simulink model "Model_6DOF_B3"  (R2020b)
settings: Solver=FixedStepAuto  StartTime=0.0  StopTime=120  FixedStep=0.05  RelTol=1e-3
values from neighbouring files (symbols this model uses):
  Ba_0 = [0 0 0 0 0 0]    [ctrl_mode_param.m]
  Bb = 4418825.3321    [load_data.m]
  Bv_0 = [tgt_speed 0 0 0 0 0]    [ctrl_mode_param.m]
  Bx_0 = [0 0 tgt_depth 0 0 0]    [ctrl_mode_param.m]
  Ixx = 5.23e7    (= 52300000)    [load_data.m]
  Ixy = 0    [load_data.m]
  Ixz = 0    [load_data.m]
  Iyy = 1.375e9    (= 1375000000)    [load_data.m]
  Iyz = 0    [load_data.m]
  Izz = 1.367e9    (= 1367000000)    [load_data.m]
  Mb = 4418825.3321    [load_data.m]
  Xb = 0    [load_data.m]
  Xg = 0    [load_data.m]
  Yb = 0    [load_data.m]
  Yg = 0    [load_data.m]
  Zb = 0.4406    [load_data.m]
  Zg = 0    [load_data.m]
undefined symbols (not defined in the file or in its folder): dA_BP1, dA_BP2, dA_Hull, dA_PH, dA_Sail, dA_SProot, dA_X1a, dA_X1b, dA_X2a, dA_X2b, dA_X3a, dA_X3b, dA_X4a, dA_X4b, its, n_BP1, n_BP2, n_Hull, n_PH, n_Sail, n_SProot, n_X1a, n_X1b, n_X2a, n_X2b, n_X3a, n_X3b, n_X4a, n_X4b, nt_BP1, nt_BP2, nt_Hull, nt_PH, nt_Sail, nt_SProot, nt_X1a, nt_X1b, nt_X2a, nt_X2b, nt_X3a, nt_X3b, nt_X4a, nt_X4b, Usp, vt1_BP1, vt1_BP2, vt1_Hull, vt1_PH, vt1_Sail, vt1_SProot, vt1_X1a, vt1_X1b, vt1_X2a, vt1_X2b, vt1_X3a, vt1_X3b, vt1_X4a, vt1_X4b, vt2_BP1, vt2_BP2 ... (+27)
libraries: simulink x5
(part 11 of 15)

== matlab function Model_6DOF_B3/HDM B3/Wave, Virtual Mass and Hydrostatic/Wave Particle Motions/Subsystem/Subsystem/MATLAB Function4 ==
  data: time input; Xearth input; Fx_total output; vert1 input; vert2 input; vert3 input; dA input; ntri input; normal input; A_wave input; k_wave input; w_wave input; rho input; g input; Fy_total output; Fz_total output; Mx_total output; My_total output; Mz_total output; Zb input; its input; fwrite input
function [Fx_total,Fy_total,Fz_total,Mx_total,My_total,Mz_total]= fcn(time,Xearth,vert1,vert2,vert3,dA,ntri,normal,A_wave,k_wave,w_wave,rho,g,Zb,its,fwrite)
x_e=Xearth(1); y_e=Xearth(2); z_e=Xearth(3);
phi=Xearth(4); theta=Xearth(5); psi=Xearth(6);

RMat=[cos(theta)*cos(psi) -cos(phi)*sin(psi)+sin(phi)*sin(theta)*cos(psi)  sin(phi)*sin(psi)+cos(phi)*sin(theta)*cos(psi); ...
      cos(theta)*sin(psi)  cos(phi)*cos(psi)+sin(phi)*sin(theta)*sin(psi) -sin(phi)*cos(psi)+cos(phi)*sin(theta)*sin(psi); ...
     -sin(theta)                             sin(phi)*cos(theta)                             cos(phi)*cos(theta)];  

%position of mid points in earth coordinate;
mp1=zeros(ntri,3);
mp2=zeros(ntri,3);
mp3=zeros(ntri,3);
nA =zeros(ntri,3);

P1=zeros(ntri,1);
P2=zeros(ntri,1);
P3=zeros(ntri,1);

%position vector of mid points from the CG
r1=zeros(ntri,3);
r2=zeros(ntri,3);
r3=zeros(ntri,3);
v1_w=zeros(ntri,3);
v2_w=zeros(ntri,3);
v3_w=zeros(ntri,3);
n_w=zeros(ntri,3);

%Area of triangle, product of area and unit normal, position vector to each mid-point
for i=1:ntri
    %Area of each triangle
    A=[vert2(i,1)-vert1(i,1); vert2(i,2)-vert1(i,2); vert2(i,3)-vert1(i,3);];
    B=[vert3(i,1)-vert1(i,1); vert3(i,2)-vert1(i,2); vert3(i,3)-vert1(i,3);];
    C=[normal(i,1); normal(i,2); normal(i,3);];
        
    %A*n vector calculation
    for j=1:3
        nA(i,j)=dA(i).*C(j);    
    end
    
    %position vector to each mid point of each edge
    for j=1:3
        r1(i,j)=0.5*(vert1(i,j)+vert2(i,j));
        r2(i,j)=0.5*(vert1(i,j)+vert3(i,j));
        r3(i,j)=0.5*(vert2(i,j)+vert3(i,j));
    end
end

%computing mid point location between vertices in earth coordinate
for i=1:ntri
    MP1=RMat*[r1(i,1); r1(i,2); r1(i,3);]+[x_e; y_e; z_e;];
    MP2=RMat*[r2(i,1); r2(i,2); r2(i,3);]+[x_e; y_e; z_e;];
    MP3=RMat*[r3(i,1); r3(i,2); r3(i,3);]+[x_e; y_e; z_e;];
    
    v1i=RMat*[vert1(i,1); vert1(i,2); vert1(i,3);]+[x_e; y_e; z_e;];
    v2i=RMat*[vert2(i,1); vert2(i,2); vert2(i,3);]+[x_e; y_e; z_e;];
    v3i=RMat*[vert3(i,1); vert3(i,2); vert3(i,3);]+[x_e; y_e; z_e;];
   
    for j=1:3
        v1_w(i,j)=v1i(j); v2_w(i,j)=v2i(j); v3_w(i,j)=v3i(j); 
        mp1(i,j)=MP1(j);  mp2(i,j)=MP2(j);  mp3(i,j)=MP3(j);
    end
end

for i=1:ntri
    A=[v2_w(i,1)-v1_w(i,1); v2_w(i,2)-v1_w(i,2); v2_w(i,3)-v1_w(i,3);];
    B=[v3_w(i,1)-v1_w(i,1); v3_w(i,2)-v1_w(i,2); v3_w(i,3)-v1_w(i,3);];
    n=cross(A,B)/norm(cross(A,B));
    dA(i,1)=0.5*norm(cross(A,B));
    n_w(i,1)=n(1); n_w(i,2)=n(2); n_w(i,3)=n(3);
end

if fwrite==1
if rem(time,its)==0
%writing the transformed surface grid
filename=['./SurfOut/Hull_' sprintf('%08.2f',time) '.stl'];
fileID = fopen(filename,'w');
formatSpec='solid\n'; fprintf(fileID,formatSpec);
for i=1:ntri
fprintf(fileID,'facet normal ');
formatSpec='%1.8e %1.8e %1.8e\n';
fprintf(fileID,formatSpec,normal(i,1),normal(i,2),normal(i,3));
    fprintf(fileID,'  outer loop\n')
    fprintf(fileID,'    vertex   ')
    fprintf(fileID,formatSpec,v1_w(i,1)/70.2,v1_w(i,2)/70.2,v1_w(i,3)/70.2)
    fprintf(fileID,'    vertex   ')
    fprintf(fileID,formatSpec,v2_w(i,1)/70.2,v2_w(i,2)/70.2,v2_w(i,3)/70.2)
    fprintf(fileID,'    vertex   ')
    fprintf(fileID,formatSpec,v3_w(i,1)/70.2,v3_w(i,2)/70.2,v3_w(i,3)/70.2)
    fprintf(fileID,'  endloop\n')
    fprintf(fileID,'endfacet\n')
end
formatSpec='endsolid'; fprintf(fileID,formatSpec);
fclose(fileID);
end
end

%computing forces and moments for each triangle
Fx_total=0; Fy_total=0; Fz_total=0;
Mx_total=0; My_total=0; Mz_total=0;

for i=1:ntri
    p1=-rho*g*(mp1(i,3)-A_wave*exp(k_wave.*mp1(i,3)).*sin(k_wave*mp1(i,1)-w_wave.*time));
    p2=-rho*g*(mp2(i,3)-A_wave*exp(k_wave.*mp2(i,3)).*sin(k_wave*mp2(i,1)-w_wave.*time));
    p3=-rho*g*(mp3(i,3)-A_wave*exp(k_wave.*mp3(i,3)).*sin(k_wave*mp3(i,1)-w_wave.*time));
    
    dFx=-nA(i,1)*(p1+p2+p3)./3;
    dFy=-nA(i,2)*(p1+p2+p3)./3;
    dFz=-nA(i,3)*(p1+p2+p3)./3;
    
    dP =-p1.*[r1(i,1); r1(i,2); r1(i,3)-Zb;]...
        -p2.*[r2(i,1); r2(i,2); r2(i,3)-Zb;]...
        -p3.*[r3(i,1); r3(i,2); r3(i,3)-Zb;];
    N =[nA(i,1); nA(i,2); nA(i,3);];
    dM=cross(dP,N);
    Fx_total=Fx_total+dFx;
    Fy_total=Fy_total+dFy;
    Fz_total=Fz_total+dFz;
    Mx_total=Mx_total+dM(1)/3;
    My_total=My_total+dM(2)/3;
    Mz_total=Mz_total+dM(3)/3;
end
end

== matlab function Model_6DOF_B3/HDM B3/Wave, Virtual Mass and Hydrostatic/Wave Particle Motions/Subsystem/X1/MATLAB Function1 ==
  data: time input; Xearth input; Fx_total output; vert1 input; vert2 input; vert3 input; dA input; ntri input; normal input; A_wave input; k_wave input; w_wave input; rho input; g input; Fy_total output; Fz_total output; Mx_total output; My_total output; Mz_total output; Zb input; EAX input; dX input; its input; origin input; xcg input; fwrite input
function [Fx_total,Fy_total,Fz_total,Mx_total,My_total,Mz_total]= fcn(time,Xearth,vert1,vert2,vert3,dA,ntri,normal,A_wave,k_wave,w_wave,rho,g,Zb,EAX,dX,its,origin,xcg,fwrite)
%EAX=Appendage eulater angle in local coordinate
%its=number of time steps to skip writing grid

x_e=Xearth(1); y_e=Xearth(2); z_e=Xearth(3);
phi=Xearth(4); theta=Xearth(5); psi=Xearth(6);
phiX=EAX(1); thetaX=EAX(2); psiX=EAX(3);


RMat=[cos(theta)*cos(psi) -cos(phi)*sin(psi)+sin(phi)*sin(theta)*cos(psi)  sin(phi)*sin(psi)+cos(phi)*sin(theta)*cos(psi); ...
      cos(theta)*sin(psi)  cos(phi)*cos(psi)+sin(phi)*sin(theta)*sin(psi) -sin(phi)*cos(psi)+cos(phi)*sin(theta)*sin(psi); ...
     -sin(theta)                             sin(phi)*cos(theta)                             cos(phi)*cos(theta)];  
RMATX=[cos(thetaX)*cos(psiX) -cos(phiX)*sin(psiX)+sin(phiX)*sin(thetaX)*cos(psiX)  sin(phiX)*sin(psiX)+cos(phiX)*sin(thetaX)*cos(psiX); ...
      cos(thetaX)*sin(psiX)  cos(phiX)*cos(psiX)+sin(phiX)*sin(thetaX)*sin(psiX) -sin(phiX)*cos(psiX)+cos(phiX)*sin(thetaX)*sin(psiX); ...
     -sin(thetaX)                             sin(phiX)*cos(thetaX)                             cos(phiX)*cos(thetaX)];  
RMATD=[cos(0)*cos(dX) -cos(0)*sin(dX)+sin(0)*sin(0)*cos(dX)  sin(0)*sin(dX)+cos(0)*sin(0)*cos(dX); ...
      cos(0)*sin(dX)  cos(0)*cos(dX)+sin(0)*sin(0)*sin(dX) -sin(0)*cos(dX)+cos(0)*sin(0)*sin(dX); ...
     -sin(0)                             sin(0)*cos(0)                             cos(0)*cos(0)];  


%Rotating the vertices to put in ship coordinate
for i=1:ntri 
    V1=[vert1(i,1); vert1(i,2); vert1(i,3);];
    V2=[vert2(i,1); vert2(i,2); vert2(i,3);];
    V3=[vert3(i,1); vert3(i,2); vert3(i,3);];
        
    %rotating to local z coordinate
    V1_o=inv(RMATX)*(V1-origin*70.2+xcg);
    V2_o=inv(RMATX)*(V2-origin*70.2+xcg);
    V3_o=inv(RMATX)*(V3-origin*70.2+xcg);
    
    %rotating for corresponding appendage deflection
    V1_x=RMATD*V1_o;
    V2_x=RMATD*V2_o;
    V3_x=RMATD*V3_o;
    
        %re-positioning the appendage to local vectors
    V1_r=RMATX*V1_x;
    V2_r=RMATX*V2_x;
    V3_r=RMATX*V3_x;
    
    %re-assigning vertices
    
    for j=1:3
    vert1(i,j)=V1_r(j)+origin(j)*70.2-xcg(j);
    vert2(i,j)=V2_r(j)+origin(j)*70.2-xcg(j);
    vert3(i,j)=V3_r(j)+origin(j)*70.2-xcg(j);
    end  
end

 
%position of mid points in earth coordinate;
mp1=zeros(ntri,3);
mp2=zeros(ntri,3);
mp3=zeros(ntri,3);
nA =zeros(ntri,3);

P1=zeros(ntri,1);
P2=zeros(ntri,1);
P3=zeros(ntri,1);

%position vector of mid points from the CG
r1=zeros(ntri,3);
r2=zeros(ntri,3);
r3=zeros(ntri,3);

v1_w=zeros(ntri,3);
v2_w=zeros(ntri,3);
v3_w=zeros(ntri,3);
n_w=zeros(ntri,3);

%Area of triangle, product of area and unit normal, position vector to each mid-point

for i=1:ntri
    %Area of each triangle
    A=[vert2(i,1)-vert1(i,1); vert2(i,2)-vert1(i,2); vert2(i,3)-vert1(i,3);];
    B=[vert3(i,1)-vert1(i,1); vert3(i,2)-vert1(i,2); vert3(i,3)-vert1(i,3);];
    C=[normal(i,1); normal(i,2); normal(i,3);];

    
    %A*n vector calculation
    for j=1:3
        nA(i,j)=dA(i).*C(j);    
    end
    
    %position vector to each mid point of each edge
    for j=1:3
        r1(i,j)=0.5*(vert1(i,j)+vert2(i,j));
        r2(i,j)=0.5*(vert1(i,j)+vert3(i,j));
        r3(i,j)=0.5*(vert2(i,j)+vert3(i,j));
    end
end

%computing mid point location between vertices in earth coordinate
for i=1:ntri
    MP1=RMat*[r1(i,1); r1(i,2); r1(i,3);]+[x_e; y_e; z_e;];
    MP2=RMat*[r2(i,1); r2(i,2); r2(i,3);]+[x_e; y_e; z_e;];
    MP3=RMat*[r3(i,1); r3(i,2); r3(i,3);]+[x_e; y_e; z_e;];
    
    v1i=RMat*[vert1(i,1); vert1(i,2); vert1(i,3);]+[x_e; y_e; z_e;];
    v2i=RMat*[vert2(i,1); vert2(i,2); vert2(i,3);]+[x_e; y_e; z_e;];
    v3i=RMat*[vert3(i,1); vert3(i,2); vert3(i,3);]+[x_e; y_e; z_e;];
    
    for j=1:3
        v1_w(i,j)=v1i(j); v2_w(i,j)=v2i(j); v3_w(i,j)=v3i(j);
        mp1(i,j)=MP1(j);  mp2(i,j)=MP2(j);  mp3(i,j)=MP3(j);
    end
end

for i=1:ntri
    A=[v2_w(i,1)-v1_w(i,1); v2_w(i,2)-v1_w(i,2); v2_w(i,3)-v1_w(i,3);];
    B=[v3_w(i,1)-v1_w(i,1); v3_w(i,2)-v1_w(i,2); v3_w(i,3)-v1_w(i,3);];
    n=cross(A,B)/norm(cross(A,B));
    dA(i,1)=0.5*norm(cross(A,B));
    n_w(i,1)=n(1); n_w(i,2)=n(2); n_w(i,3)=n(3);
end

if fwrite==1
if rem(time,its)==0
%writing the transformed surface grid
filename=['./SurfOut/X1_2_' sprintf('%08.2f',time) '.stl'];
fileID = fopen(filename,'w');
formatSpec='solid\n'; fprintf(fileID,formatSpec);
for i=1:ntri
fprintf(fileID,'facet normal ');
formatSpec='%1.8e %1.8e %1.8e\n';
fprintf(fileID,formatSpec,normal(i,1),normal(i,2),normal(i,3));
    fprintf(fileID,'  outer loop\n')
    fprintf(fileID,'    vertex   ')
    fprintf(fileID,formatSpec,v1_w(i,1)/70.2,v1_w(i,2)/70.2,v1_w(i,3)/70.2)
    fprintf(fileID,'    vertex   ')
    fprintf(fileID,formatSpec,v2_w(i,1)/70.2,v2_w(i,2)/70.2,v2_w(i,3)/70.2)
    fprintf(fileID,'    vertex   ')
    fprintf(fileID,formatSpec,v3_w(i,1)/70.2,v3_w(i,2)/70.2,v3_w(i,3)/70.2)
    fprintf(fileID,'  endloop\n')
    fprintf(fileID,'endfacet\n')
end
formatSpec='endsolid'; fprintf(fileID,formatSpec);
fclose(fileID);
end
end

%computing forces and moments for each triangle
Fx_total=0; Fy_total=0; Fz_total=0;
Mx_total=0; My_total=0; Mz_total=0;

for i=1:ntri
    p1=-rho*g*(mp1(i,3)-A_wave*exp(k_wave.*mp1(i,3)).*sin(k_wave*mp1(i,1)-w_wave.*time));
    p2=-rho*g*(mp2(i,3)-A_wave*exp(k_wave.*mp2(i,3)).*sin(k_wave*mp2(i,1)-w_wave.*time));
    p3=-rho*g*(mp3(i,3)-A_wave*exp(k_wave.*mp3(i,3)).*sin(k_wave*mp3(i,1)-w_wave.*time));
    
    dFx=-nA(i,1)*(p1+p2+p3)./3;
    dFy=-nA(i,2)*(p1+p2+p3)./3;
    dFz=-nA(i,3)*(p1+p2+p3)./3;
    
    dP =-p1.*[r1(i,1); r1(i,2); r1(i,3)-Zb;]...
        -p2.*[r2(i,1); r2(i,2); r2(i,3)-Zb;]...
        -p3.*[r3(i,1); r3(i,2); r3(i,3)-Zb;];
    N =[nA(i,1); nA(i,2); nA(i,3);];
    dM=cross(dP,N);
    Fx_total=Fx_total+dFx;
    Fy_total=Fy_total+dFy;
    Fz_total=Fz_total+dFz;
    Mx_total=Mx_total+dM(1)/3;
    My_total=My_total+dM(2)/3;
    Mz_total=Mz_total+dM(3)/3;
end
end

== matlab function Model_6DOF_B3/HDM B3/Wave, Virtual Mass and Hydrostatic/Wave Particle Motions/Wave Properties ==
  data: SeaState input; L_wave output; A_wave output; k_wave output; w_wave output
function [L_wave,A_wave,k_wave,w_wave] = fcn(SeaState)

   if SeaState==2;
       L_wave= 87.8; A_wave= 0.15;
   elseif SeaState==3;
       L_wave= 87.8; A_wave= 0.44;
   elseif SeaState==4;
       L_wave= 120.9; A_wave= 0.94;
   elseif SeaState==5;
       L_wave= 140.9; A_wave= 1.625;
   elseif SeaState==6;
       L_wave=240.1; A_wave=2.5;
   elseif SeaState==7;
       L_wave= 351.3; A_wave= 3.750;
   else
       L_wave= 0; A_wave=0;
   end
   
   if(L_wave==0)
       k_wave=0;
   else
       k_wave=2*pi/L_wave;
   end
   
   w_wave=sqrt(9.81*k_wave);
   
end

== matlab function Model_6DOF_B3/HDM B3/Wave, Virtual Mass and Hydrostatic/Wave Particle Motions/Wave particle velocity at hull CG ==
  data: time input; X_earth input; uwsCG output; dLCG input; L_wave input; phi_wave input; beta_wave input; A_wave input; k_wave input; w_wave input; uweCG output
function [uwsCG,uweCG] = fcn(time,X_earth,dLCG,L_wave,phi_wave,beta_wave,A_wave,k_wave,w_wave)
 
    Xs=[X_earth(1); X_earth(2); X_earth(3);];
    phi= X_earth(4); theta= X_earth(5); psi= X_earth(6); % Euler angles
    
    RMat=[cos(theta)*cos(psi) -cos(phi)*sin(psi)+sin(phi)*sin(theta)*cos(psi)  sin(phi)*sin(psi)+cos(phi)*sin(theta)*cos(psi); ...
          cos(theta)*sin(psi)  cos(phi)*cos(psi)+sin(phi)*sin(theta)*sin(psi) -sin(phi)*cos(psi)+cos(phi)*sin(theta)*sin(psi); ...
        -sin(theta)                             sin(phi)*cos(theta)                             cos(phi)*cos(theta)];  

    u_w=-A_wave*w_wave*exp(k_wave*Xs(3))*cos(k_wave*Xs(1)-w_wave*time+phi_wave)*cos(pi*beta_wave);
    v_w= A_wave*w_wave*exp(k_wave*Xs(3))*cos(k_wave*Xs(1)-w_wave*time+phi_wave)*sin(pi*beta_wave);
    w_w=-A_wave*w_wave*exp(k_wave*Xs(3))*sin(k_wave*Xs(1)-w_wave*time+phi_wave);
    
    uweCG = [u_w; v_w; w_w;];
    uwsCG = inv(RMat)*uweCG;
    
end

== matlab function Model_6DOF_B3/HDM B3/X/Fx ==
  data: Bx input; Bv input; Ba input; CXqq input; CXuvwV input; CXuvwH input; Umag input; dLCG input; dmass input; UeSP input; XdXi input; X output; Tprop input; Mb parameter; Bb parameter; Xvm input; Xapp output; Xhull output; Tout output; X_Hyd output; XdX output; BFX input; Xstat output
function [X,Xapp,Xhull,Tout,X_Hyd,XdX,Xstat]   = fcn(Bx,Bv,Ba,CXqq,CXuvwV,CXuvwH,Umag,dLCG,dmass,UeSP,XdXi,Tprop,Mb,Bb,Xvm,BFX)
%Bx,Bv,Ba are the body motion position, velocity, acceleration in ship coordinate
%Wv,Wa are the wave particle velocity, acceleration in ship coordinate

u=Bv(1); v=Bv(2); w=Bv(3); p=Bv(4); q=Bv(5); r=Bv(6);
x=Bx(1); y=Bx(2); z=Bx(3); phi=Bx(4); theta=Bx(5); psi=Bx(6);
a1=Ba(1); a2=Ba(2); a3=Ba(3); a4=Ba(4); a5=Ba(5); a6=Ba(6); 

%Xwq=1025*70.2^3*CXwq
%Twq=0.5*1025*70.2^3*CTwq
%Xstat=BFX-(Mb+dmass)*9.81*sin(Bx(5));%-((Mb+dmass)-Bb)*9.81*sin(Bx(5));

Xqq=0.5*1025*70.2^4*q^2*CXqq;
Xwq=1025*70.2^3*(-3.3124286E-03*w*q)
Xvr=1025*70.2^3*(-3.3124286E-03*v*r)*0
Twq=0.5*1025*70.2^3*(3.6594E-03*w*q)
Tvr=0.5*1025*70.2^3*(3.6594E-03*v*r)*0

dXiuq=(4.4603E-03*(u*q)^2-7.3687E-06*(u*q))


XX1=0.5*1025*70.2^2*(XdXi(1)+dXiuq)*UeSP(1)^2
XX2=0.5*1025*70.2^2*(XdXi(2)+dXiuq)*UeSP(2)^2
XX3=0.5*1025*70.2^2*(XdXi(3)+dXiuq)*UeSP(3)^2
XX4=0.5*1025*70.2^2*(XdXi(4)+dXiuq)*UeSP(4)^2
XXB=0.5*1025*(70.2^2*XdXi(5)*UeSP(5)^2)

XdX=[XX1; XX2; XX3; XX4; XXB;]

Xapp=XX1+XX2+XX3+XX4+XXB;
Xuvw=-0.5*1025*70.2^2*(CXuvwV+CXuvwH)*Umag^2*u/abs(u);
Xstat=BFX+(Mb+dmass)*9.81*sin(Bx(5))
Xhull=Xqq+Xuvw+Xwq+Xvr;
Tout=Tprop+Twq+Tvr;
X_Hyd=Xapp+Xhull+Xstat-Tout;
X=Xapp+Xhull+Xstat-Tout+Xvm;

== matlab function Model_6DOF_B3/HDM 6DOF V1/Effective Veloicity Calclation/MATLAB Function1 ==
  data: rX1 input; urX1 output; rX2 input; urX2 output; urX3 output; urX4 output; urXB output; rX3 input; rX4 input; rXB input; U_ship input
function [urX1,urX2,urX3,urX4,urXB]= fcn(rX1,rX2,rX3,rX4,rXB,U_ship)

%rXi: position vector of Stern planes from the CG
%rXB: position vector of sail planes from the CG
%U_ship: rigid body velcity in the ship system

u_ship=[U_ship(1); U_ship(2); U_ship(3);]
w_ship=[U_ship(4); U_ship(5); U_ship(6);]

urX1=-u_ship+cross(rX1,w_ship);
urX2=-u_ship+cross(rX2,w_ship);
urX3=-u_ship+cross(rX3,w_ship);
urX4=-u_ship+cross(rX4,w_ship);
urXB=-u_ship+cross(rXB,w_ship);

end

== matlab function Model_6DOF_B3/HDM B1/Effective Veloicity Calclation/MATLAB Function ==
  data: nh input; n1 input; aX output; n2 input; n3 input; n4 input; nB input; urX1 input; urX2 input; urX3 input; urX4 input; urXB input; UeX output
function [aX,UeX] = fcn(nh,n1,n2,n3,n4,nB,urX1,urX2,urX3,urX4,urXB)

%urXi: relative velocity of rigid body motion and wave particle velocity to the ith stern plane
%ni  : base vector of i-th plane's axis direction
%nh  : base vector of the hull axis direction
IP=zeros(5,1); %IP determines the sign of the angle of attack. if the dot product is negative, angle is greater than 90degs.
aX=zeros(5,1);

np1=dot(nh,urX1)*nh+dot(n1,urX1)*n1;
np2=dot(nh,urX2)*nh+dot(n2,urX2)*n2;
np3=dot(nh,urX3)*nh+dot(n3,urX3)*n3;
np4=dot(nh,urX4)*nh+dot(n4,urX4)*n4;
npB=dot(nh,urXB)*nh+dot(nB,urXB)*nB;

arg1=dot(np1,urX1)/(norm(np1)*norm(urX1));
arg2=dot(np2,urX2)/(norm(np2)*norm(urX2));
arg3=dot(np3,urX3)/(norm(np3)*norm(urX3));
arg4=dot(np4,urX4)/(norm(np4)*norm(urX4));
arg5=dot(npB,urXB)/(norm(npB)*norm(urXB));

%to prevent numerical error: acos returns complex solution. used if statement
if arg1 >=1
   aX(1,1)=0;
else
   aX(1,1)=acos(arg1)*180/pi*sqrt(2);
end

if arg2 >=1
   aX(2,1)=0;
else
   aX(2,1)=acos(arg2)*180/pi*sqrt(2);
end

if arg3 >=1
   aX(3,1)=0;
else
   aX(3,1)=acos(arg3)*180/pi*sqrt(2);
end

if arg4 >=1
   aX(4,1)=0;
else
   aX(4,1)=acos(arg4)*180/pi*sqrt(2);
end

if arg5 >=1
   aX(5,1)=0;
else
   aX(5,1)=acos(arg5)*180/pi;
end

d1=cross(n1,nh);
d2=cross(n2,nh);
d3=cross(n3,nh);
d4=cross(n4,nh);
dB=cross(nB,nh);

IP(1,1)=dot(d1,urX1);
IP(2,1)=dot(d2,urX2);
IP(3,1)=dot(d3,urX3);
IP(4,1)=dot(d4,urX4);
IP(5,1)=dot(dB,urXB);

for i=1:5
    if IP(i,1)<0
        aX(i,1)=-aX(i,1)
    end
end    

UeX=[norm(urX1); norm(urX2); norm(urX3); norm(urX4); norm(urXB);];
end

== matlab function Model_6DOF_B3/HDM B1/Effective Veloicity Calclation/MATLAB Function1 ==
  data: rX1 input; urX1 output; rX2 input; urX2 output; urX3 output; urX4 output; urXB output; rX3 input; rX4 input; rXB input; U_ship input
function [urX1,urX2,urX3,urX4,urXB]= fcn(rX1,rX2,rX3,rX4,rXB,U_ship)

%rXi: position vector of Stern planes from the CG
%rXB: position vector of sail planes from the CG
%U_ship: rigid body velcity in the ship system

u_ship=[U_ship(1); U_ship(2); U_ship(3);]
w_ship=[U_ship(4); U_ship(5); U_ship(6);]

urX1=-u_ship+cross(rX1,w_ship);
urX2=-u_ship+cross(rX2,w_ship);
urX3=-u_ship+cross(rX3,w_ship);
urX4=-u_ship+cross(rX4,w_ship);
urXB=-u_ship+cross(rXB,w_ship);

end

== matlab function Model_6DOF_B3/HDM B1/Effective Veloicity Calclation/MATLAB Function2 ==
  data: Bv input; alpha output; beta output; Umag output; uCG input; vCG input; wCG input
function [alpha,beta,Umag] = fcn(Bv,uCG,vCG,wCG)

    u_eff=uCG-Bv(1);
    v_eff=vCG-Bv(2);
    w_eff=wCG-Bv(3);
    
    U_eff=[u_eff; v_eff; w_eff;];
    
    if abs(u_eff) <= 1e-8
        alpha=90; beta=90;
        if v_eff < 0
            beta = -90;
        end
        if w_eff < 0
            alpha = -90;
        end
    else
        beta  = -atan(v_eff/u_eff)*180/pi;
        alpha =  atan(w_eff/u_eff)*180/pi;
    end
    
    Umag =norm(U_eff);
end

== matlab function Model_6DOF_B3/HDM B1/K/Mx ==
  data: Bx input; Bv input; Ba input; CKup input; CKur input; CKpp input; CKuvw input; Umag input; UeX input; dLCG input; dmass input; CNdXi input; K output; KApp output; K_hull output; Xg parameter; Bb parameter; Xb parameter; Mb parameter; Zg parameter; Zb parameter; Kh_total output; Kpp output; Kvm input; KAppAll output; BFK input; KStat output; KHullVM output
function [K,KApp,K_hull,Kh_total,Kpp,KAppAll,KStat,KHullVM]  = fcn(Bx,Bv,Ba, CKup,CKur,CKpp,CKuvw,Umag,UeX,dLCG,dmass,CNdXi,Xg,Bb,Xb,Mb,Zg,Zb,Kvm,BFK)
%Bx,Bv,Ba are the body motion position, velocity, acceleration in ship coordinate
%Wv,Wa are the wave particle velocity, acceleration in ship coordinate

u=Bv(1); v=Bv(2); w=Bv(3); p=Bv(4); q=Bv(5); r=Bv(6);
x=Bx(1); y=Bx(2); z=Bx(3); phi=Bx(4); theta=Bx(5); psi=Bx(6);
a1=Ba(1); a2=Ba(2); a3=Ba(3); a4=Ba(4); a5=Ba(5); a6=Ba(6); 

KdX1=70.2^3*1025*CNdXi(1)*UeX(1)^2;
KdX2=70.2^3*1025*CNdXi(2)*UeX(2)^2;
KdX3=70.2^3*1025*CNdXi(3)*UeX(3)^2;
KdX4=70.2^3*1025*CNdXi(4)*UeX(4)^2;

Kup = -70.2^3*1025*(-2.9648E-04*u*p)*u^2;
Kur = 70.2^3*1025*(-5.6192E-05*u*r)*u^2;
Kpp = 70.2^3*1025*(-1.0622E-01*p*abs(p));
Kuvw=0.5*70.2^3*1025*CKuvw*Umag^2;

KAppAll=[KdX1; KdX2; KdX3; KdX4;]

K_hull=Kuvw+Kup+Kur+Kpp;
KHullVM=K_hull+Kvm;
KApp=KdX1+KdX2+KdX3+KdX4;
KStat= (Xg*(Mb+dmass))*cos(theta)*sin(phi)+BFK%(Xg*(Mb+dmass)-Xb*Bb)*cos(theta)*sin(phi);
%Kstat needs to be checked for the mass term's sign
Kh_total=K_hull+KApp+KStat+Kpp
K=K_hull+KApp+KStat+Kvm+Kpp;
end

== matlab function Model_6DOF_B3/HDM B1/M/My ==
  data: Bx input; Bv input; Ba input; Mqq input; Mwq input; Mprop input; Muvw input; Umag input; UeSP input; dLCG input; dmass input; MdXi input size=5; MY output; Xg parameter; Bb parameter; Xb parameter; Mb parameter; Zg parameter; Zb parameter; Mvm input; MYApp output; MYStat output; Mprop output; M_hull output; MY_hyd output; MYApp_All output; BFM input
function [MY, MYApp, MYStat, Mprop, M_hull,MY_hyd,MYApp_All] = fcn(Bx,Bv,Ba,Mqq,Mwq,Mprop,Muvw,Umag,UeSP,dLCG,dmass,MdXi,Xg,Bb,Xb,Mb,Zg,Zb,Mvm,BFM)
%wqfunction [MY,MYApp,MYStat,Mprop,M_hull]  = fcn(Bx,Bv,Ba,Mqq,Mwq,Muq,Mprop,Muvw,Umag,UeSP,dLCG,dmass,MdXi,Xg,Bb,Xb,Mb,Zg,Zb,Mvm,M_ext)
%Bx,Bv,Ba are the body motion position, velocity, acceleration in ship coordinate
%Wv,Wa are the wave particle velocity, acceleration in ship coordinate

u=Bv(1); v=Bv(2); w=Bv(3); p=Bv(4); q=Bv(5); r=Bv(6);
x=Bx(1); y=Bx(2); z=Bx(3); phi=Bx(4); theta=Bx(5); psi=Bx(6);
a1=Ba(1); a2=Ba(2); a3=Ba(3); a4=Ba(4); a5=Ba(5); a6=Ba(6); 

%MYuq=0.5*70.2^4*1025*Muq
%MYStat=Bb*9.81*dLCG*cos(theta)-Bb*9.81*(Zb-Zg)*sin(theta);

MYX1=0.5*70.2^3*1025*MdXi(1)*UeSP(1)^2;
MYX2=0.5*70.2^3*1025*MdXi(2)*UeSP(2)^2;
MYX3=0.5*70.2^3*1025*MdXi(3)*UeSP(3)^2;
MYX4=0.5*70.2^3*1025*MdXi(4)*UeSP(4)^2;
MYXb=0.5*70.2^3*1025*MdXi(5)*UeSP(5)^2;

MYApp_All=[MYX1; MYX2; MYX3; MYX4; MYXb;];

MYStat= BFM;
MYqq=0.5*70.2^5*1025*Mqq*q*abs(q);
MYuq=0.5*70.2^4*1025*u*q*1.9444E-03*1.1;

MYwq=0.5*70.2^4*1025*Mwq*w*abs(q);
MYuvw=0.5*70.2^3*1025*Muvw*Umag^2;
MYApp=(MYX1+MYX2+MYX3+MYX4+MYXb)*1;
Mprop=-1025*70.2^4*u*q*Mprop;

M_hull=MYuvw+MYuq;
MY_hyd=MYApp+MYStat+Mprop+M_hull;
MY=MYApp+MYStat+Mprop+M_hull+Mvm;
end

== matlab function Model_6DOF_B3/HDM B1/M 6d org/MATLAB Function2 ==
  data: u input; y output
function y = fcn(u)

y = abs(u);

== matlab function Model_6DOF_B3/HDM B1/M 6d org/My ==
  data: Bx input; Bv input; Ba input; Mqq input; Mwq input; Muq input; Mprop input; Muvw input; Umag input; UeX input; dLCG input; dmass input; MdXi input; MY output; Xg parameter; Bb parameter; Xb parameter; Mb parameter; Zg parameter; Zb parameter; Mvm input; MYApp output; MYStat output; MYhull output; MYprop output
function [MY,MYApp,MYStat,MYhull,MYprop]   = fcn(Bx,Bv,Ba,Mqq,Mwq,Muq,Mprop,Muvw,Umag,UeX,dLCG,dmass,MdXi,Xg,Bb,Xb,Mb,Zg,Zb,Mvm)
%Bx,Bv,Ba are the body motion position, velocity, acceleration in ship coordinate
%Wv,Wa are the wave particle velocity, acceleration in ship coordinate

u=Bv(1); v=Bv(2); w=Bv(3); p=Bv(4); q=Bv(5); r=Bv(6);
x=Bx(1); y=Bx(2); z=Bx(3); phi=Bx(4); theta=Bx(5); psi=Bx(6);
a1=Ba(1); a2=Ba(2); a3=Ba(3); a4=Ba(4); a5=Ba(5); a6=Ba(6); 

MYX1=0.5*70.2^3*1025*MdXi(1)*UeX(1)^2;
MYX2=0.5*70.2^3*1025*MdXi(2)*UeX(2)^2;
MYX3=0.5*70.2^3*1025*MdXi(3)*UeX(3)^2;
MYX4=0.5*70.2^3*1025*MdXi(4)*UeX(4)^2;
MYXb=0.5*70.2^3*1025*MdXi(5)*UeX(5)^2;

MYStat= Bb*9.81*dLCG*cos(theta)-Bb*9.81*(Zb-Zg)*sin(theta);

MYqq=0.5*70.2^5*1025*Mqq*q*abs(q);
MYuq=0.5*70.2^4*1025*Muq
MYwq=0.5*70.2^4*1025*Mwq*w*abs(q);
MYuvw=0.5*70.2^3*1025*Muvw*Umag^2;
MYApp=(MYX1+MYX2+MYX3+MYX4+MYXb);
MYprop=-1025*70.2^4*u*q*Mprop;

MYhull=MYuvw+MYuq+Mvm
MY=MYApp+MYStat+MYhull+MYprop
end

== matlab function Model_6DOF_B3/HDM 6DOF V1/M/MATLAB Function2 ==
  data: u input; y output
function y = fcn(u)

y = abs(u);

== matlab function Model_6DOF_B3/HDM B1/N/Mz ==
  data: Bx input; Bv input; Ba input; CNr input; CNrr input; CNvr input; CNuvw input; Umag input; UeX input; dLCG input; dmass input; CNdXi input; N output; NApp output; N_hull output; Xg parameter; Bb parameter; Xb parameter; Mb parameter; Zg parameter; Zb parameter; Nh_Total output; Nprop output; NStat output; NAppAll output; Nvm input; BFN input; NHullVM output; Nvr output; Nrr output; Nuvw output; Nr output
function [N,NApp,N_hull,Nh_Total,Nprop,NStat,NAppAll,NHullVM,Nvr,Nrr,Nuvw,Nr]  = fcn(Bx,Bv,Ba, CNr,CNrr,CNvr,CNuvw,Umag,UeX,dLCG,dmass,CNdXi,Xg,Bb,Xb,Mb,Zg,Zb,Nvm,BFN)
%Bx,Bv,Ba are the body motion position, velocity, acceleration in ship coordinate
%Wv,Wa are the wave particle velocity, acceleration in ship coordinate

u=Bv(1); v=Bv(2); w=Bv(3); p=Bv(4); q=Bv(5); r=Bv(6);
x=Bx(1); y=Bx(2); z=Bx(3); phi=Bx(4); theta=Bx(5); psi=Bx(6);
a1=Ba(1); a2=Ba(2); a3=Ba(3); a4=Ba(4); a5=Ba(5); a6=Ba(6); 

NdX1=70.2^3*1025*CNdXi(1)*UeX(1)^2;
NdX2=70.2^3*1025*CNdXi(2)*UeX(2)^2;
NdX3=70.2^3*1025*CNdXi(3)*UeX(3)^2;
NdX4=70.2^3*1025*CNdXi(4)*UeX(4)^2;

Nr  =0.5*70.2^3*1025*(7.6545E-03*0.8*u*r)*u^2;
%Nr  =-0.5*70.2^3*1025*CNr*u^2*3;
Nvr =0.5*70.2^3*1025*CNvr*u^2; %major source of error in it
Nrr =-0.5*70.2^3*1025*CNrr*r^2*u^2;
Nuvw=0.5*70.2^3*1025*CNuvw*Umag^2
Nprop=0.5*70.2^3*1025*u^2*(-0.0055*r)

NApp=NdX1+NdX2+NdX3+NdX4;
N_hull=Nuvw+Nr+Nvr+Nrr;
NHullVM=N_hull+Nvm
NStat= BFN%(Xg*(Mb+dmass)-Xb*Bb)*cos(theta)*sin(phi);

NAppAll=[NdX1; NdX2; NdX3; NdX4;];
Nh_Total=N_hull+NApp+NStat

N=N_hull+NApp+NStat+Nvm;
end

== matlab function Model_6DOF_B3/HDM 6DOF V1/Wave Particle Velocity/Wave Particle Motions/Sectional Position Vectors ==
  data: X_earth input; CGi input; CG input; Xce output; Rs output; dLCG input
function [Xce,Rs]  = fcn(X_earth,CGi,CG,dLCG)

%Inputs
%CGi : Volumetric center of each section.
%CG : Volumetric center of the hull in ship system. x measured from the nose, y and z measured from the shaft level.
%X_earth : Global ship position in the ship coordinate system

%Outputs
%Xce : Global position of volumetric center of each section.
%Rs  : Position vector of sectional CGs wrt the ship's CG

phi = X_earth(4); theta = X_earth(5); psi = X_earth(6);
nx=length(CGi);
Rs  = zeros(nx,3);
Xce = zeros(nx,3); 

    for i=1:nx
        for j=1:3
            Rs(i,j) = CGi(i,j)-CG(j);
        end
    end

%transformation vector using Euler angles
RMat=[cos(theta)*cos(psi) -cos(phi)*sin(psi)+sin(phi)*sin(theta)*cos(psi)  sin(phi)*sin(psi)+cos(phi)*sin(theta)*cos(psi); ...
      cos(theta)*sin(psi)  cos(phi)*cos(psi)+sin(phi)*sin(theta)*sin(psi) -sin(phi)*cos(psi)+cos(phi)*sin(theta)*sin(psi); ...
     -sin(theta)                             sin(phi)*cos(theta)                             cos(phi)*cos(theta)];
    
    for i=1:nx
        for j=1:3
            Rsi = [Rs(i,1); Rs(i,2); Rs(i,3);];
            Rei = X_earth(j) + RMat*Rsi;
            Xce(i,j) = Rei(j);
        end
    end
    
end

== matlab function Model_6DOF_B3/HDM 6DOF V1/Wave Particle Velocity/Wave Particle Motions/Wave Properties ==
  data: SeaState input; L_wave output; A_wave output; k_wave output; w_wave output
function [L_wave,A_wave,k_wave,w_wave] = fcn(SeaState)

   if SeaState==2;
       L_wave= 87.8; A_wave= 0.15;
   elseif SeaState==3;
       L_wave= 87.8; A_wave= 0.44;
   elseif SeaState==4;
       L_wave= 120.9; A_wave= 0.94;
   elseif SeaState==5;
       L_wave= 140.9; A_wave= 1.625;
   elseif SeaState==6;
       L_wave=240.1; A_wave=2.5;
   elseif SeaState==7;
       L_wave= 351.3; A_wave= 3.750;
   else
       L_wave= 0; A_wave=0;
   end
   
   if(L_wave==0)
       k_wave=0;
   else
       k_wave=2*pi/L_wave;
   end
   
   w_wave=sqrt(9.81*k_wave);
   
end

== matlab function Model_6DOF_B3/HDM 6DOF V1/Wave Particle Velocity/Wave Particle Motions/Local eff. Depth ==
  data: time input; z_eff output; Bxe input; k_wave input; w_wave input; a_wave input
function z_eff  = fcn(time,Bxe,k_wave,w_wave,a_wave)
%Regular wave is currently implemented
xe=Bxe(1); ye=Bxe(2); ze=Bxe(3); phi=Bxe(4); theta=Bxe(5); psi=Bxe(6);

elev_local=a_wave.*sin(k_wave.*xe-w_wave*time)*exp(k_wave*ze); %Check if this is identical with REX
z_eff=ze-elev_local;

end

== matlab function Model_6DOF_B3/HDM 6DOF V1/Wave Particle Velocity/Wave Particle Motions/Sectional Wave Particle & Rigid Body Velocities ==
  data: time input; U_ship input; X_earth input; Xce input; Rs input; phi_wave input; beta_wave input; Uws output; L_wave input; A_wave input; k_wave input; w_wave input; Urs output
function [Uws,Urs] = fcn(time,U_ship,X_earth,Xce,Rs,phi_wave,beta_wave,L_wave,A_wave,k_wave,w_wave)
%Inputs
%Rs      : Position vector of each sectional component in ship system.
%X_earth : Global ship position in the earth coordinate system
%U_ship  : Ship's velocity at CG in the ship coordinate system
%L, A, T, k, w of wave: wave properties for given sea state

%Outputs
%Uws: Sectional wave particle velcity vector in ship coordinate system
%Urs: Sectional rigid body translationl velocity vector in ship coordinate system

phi= X_earth(4); theta= X_earth(5); psi= X_earth(6); % Euler angles
u_s= U_ship(1); v_s=U_ship(2); w_s=U_ship(3); p_s= U_ship(4); q_s=U_ship(5); r_s=U_ship(6);

ni = length(Xce); %number, and the order of sectional elements

Uws = zeros(15,3); Urs = zeros(15,3);

Omega_s = [p_s; q_s; r_s;]; %angular velocity of the CG in ship coordinate system
Us_CG   = [u_s; v_s; w_s;]; %Translational velocity of the CG in ship coordinate system

RMat=[cos(theta)*cos(psi) -cos(phi)*sin(psi)+sin(phi)*sin(theta)*cos(psi)  sin(phi)*sin(psi)+cos(phi)*sin(theta)*cos(psi); ...
      cos(theta)*sin(psi)  cos(phi)*cos(psi)+sin(phi)*sin(theta)*sin(psi) -sin(phi)*cos(psi)+cos(phi)*sin(theta)*sin(psi); ...
     -sin(theta)                             sin(phi)*cos(theta)                             cos(phi)*cos(theta)];

%phi_wave  = 0; % wave phase. parameterized
%beta_wave = 0; % wave heading. parameterized

    for i= 1:ni
        u_w=-A_wave*w_wave*exp(k_wave*Xce(i,3))*cos(k_wave*Xce(i,1)-w_wave*time+phi_wave)*cos(pi*beta_wave);
        v_w= A_wave*w_wave*exp(k_wave*Xce(i,3))*cos(k_wave*Xce(i,1)-w_wave*time+phi_wave)*sin(pi*beta_wave);
        w_w=-A_wave*w_wave*exp(k_wave*Xce(i,3))*sin(k_wave*Xce(i,1)-w_wave*time+phi_wave);
        
        Uwe = [u_w; v_w; w_w;];
        Uint= inv(RMat)*Uwe;
        Uws(i,:) = Uint(:);  %keep Uws for further use in wave AOA calculation     
    end
    
    %Computation of translational velcity of volumetric center of sections.   
    for i=1:ni
        r_i      = [Rs(i,1); Rs(i,2); Rs(i,3)];
        Ur_int   = Us_CG + cross(r_i,Omega_s);
        for j=1:3
            Urs(i,j)=Ur_int(j); 
        end
    end
end

== matlab function Model_6DOF_B3/HDM B1/Wave, Virtual Mass and Hydrostatic/MATLAB Function ==
  data: dXm output; dYm output; dZm output; dKm output; dMm output; dNm output; cvm input; Awrs input; Rs input; Fvm output; Mvm output
function [dXm,dYm,dZm,dKm,dMm,dNm,Fvm,Mvm]  = fcn(cvm,Awrs,Rs)
%Inputs to the subroutine
%Rs  = position vector of sectional elements' CG in ship coordinate system.
%dm  = water volume mass of each section. could be replaced by the sectional volume.
%Ars = acceleration vector of each section in ship coordinate system
%Aws = sectional acceleration vector of wave particles in ship coordinate system
%cvm = sectional virtual mass coefficients. Input size is n x 3.

%Outputs from the subroutine
%Fvm  = total virtual mass force vector
%dFvm = sectional virtual mass force vector
%Mvm  = total virtual mass moment vector
%dMvm = sectional virtual mass moment vector

ni=15;%length(cvm); %number of sectional elements
dFvm = zeros(ni,3); dMvm = zeros(ni,3);
 Fvm = zeros(1,3);   Mvm = zeros(1,3);
 
 dXm=zeros(ni,1);
 dYm=zeros(ni,1);
 dZm=zeros(ni,1);
 dKm=zeros(ni,1);
 dMm=zeros(ni,1);
 dNm=zeros(ni,1);
 
%Fvm_out  = zeros(3);  Mvm_out = zeros(3); %temporary variable for report

for i=1:ni
    for j=1:3
        dFvm(i,j) = cvm(i,j)*Awrs(i,j);    
         Fvm(1,j)   = Fvm(1,j)+dFvm(i,j);   
    end
    
    Rsi   = [Rs(i,1);     Rs(i,2);   Rs(i,3);];
    dFvmi = [dFvm(i,1); dFvm(i,2); dFvm(i,3);];
    dMvmi = cross(Rsi,dFvmi);%cross(dFvmi,Rsi);
    
    for j=1:3
        dMvm(i,j) = dMvmi(j);
         Mvm(1,j) = Mvm(1,j)+dMvm(i,j);
    end
    
    for i=1:ni
        dXm(i,1)=dFvm(i,1);
        dYm(i,1)=dFvm(i,2);
        dZm(i,1)=dFvm(i,3);
        dKm(i,1)=dMvm(i,1);
        dMm(i,1)=dMvm(i,2);
        dNm(i,1)=dMvm(i,3);    
    end

  end

== matlab function Model_6DOF_B3/HDM B1/Wave, Virtual Mass and Hydrostatic/MATLAB Function1 ==
  data: awsCG input; asCG input; Fvm output; Mb parameter
function Fvm= fcn(awsCG,asCG, Mb)

Fvm=zeros(1,3);
cvm=zeros(1,3);

cvm(1,1)=0.05; cvm(1,2)=1.15; cvm(1,3)=0.81;

for i=1:3
    Fvm(i)=Mb.*cvm(1,i).*(awsCG(i)-asCG(i));
end

end

== matlab function Model_6DOF_B3/HDM B1/Wave, Virtual Mass and Hydrostatic/Wave Particle Motions/Local eff. Depth ==
  data: time input; z_eff output; Bxe input; k_wave input; w_wave input; a_wave input
function z_eff  = fcn(time,Bxe,k_wave,w_wave,a_wave)
%Regular wave is currently implemented
xe=Bxe(1); ye=Bxe(2); ze=Bxe(3); phi=Bxe(4); theta=Bxe(5); psi=Bxe(6);

elev_local=a_wave.*sin(k_wave.*xe-w_wave*time)*exp(k_wave*ze); %Check if this is identical with REX
z_eff=ze-elev_local;

end

== matlab function Model_6DOF_B3/HDM B3/Wave, Virtual Mass and Hydrostatic/Wave Particle Motions/Subsystem/X2/MATLAB Function1 ==
  data: time input; Xearth input; Fx_total output; vert1 input; vert2 input; vert3 input; dA input; ntri input; normal input; A_wave input; k_wave input; w_wave input; rho input; g input; Fy_total output; Fz_total output; Mx_total output; My_total output; Mz_total output; Zb input; EAX input; dX input; its input; origin input; xcg input; fwrite input
function [Fx_total,Fy_total,Fz_total,Mx_total,My_total,Mz_total]= fcn(time,Xearth,vert1,vert2,vert3,dA,ntri,normal,A_wave,k_wave,w_wave,rho,g,Zb,EAX,dX,its,origin,xcg,fwrite)
%EAX=Appendage eulater angle in local coordinate
%its=number of time steps to skip writing grid

x_e=Xearth(1); y_e=Xearth(2); z_e=Xearth(3);
phi=Xearth(4); theta=Xearth(5); psi=Xearth(6);
phiX=EAX(1); thetaX=EAX(2); psiX=EAX(3);


RMat=[cos(theta)*cos(psi) -cos(phi)*sin(psi)+sin(phi)*sin(theta)*cos(psi)  sin(phi)*sin(psi)+cos(phi)*sin(theta)*cos(psi); ...
      cos(theta)*sin(psi)  cos(phi)*cos(psi)+sin(phi)*sin(theta)*sin(psi) -sin(phi)*cos(psi)+cos(phi)*sin(theta)*sin(psi); ...
     -sin(theta)                             sin(phi)*cos(theta)                             cos(phi)*cos(theta)];  
RMATX=[cos(thetaX)*cos(psiX) -cos(phiX)*sin(psiX)+sin(phiX)*sin(thetaX)*cos(psiX)  sin(phiX)*sin(psiX)+cos(phiX)*sin(thetaX)*cos(psiX); ...
      cos(thetaX)*sin(psiX)  cos(phiX)*cos(psiX)+sin(phiX)*sin(thetaX)*sin(psiX) -sin(phiX)*cos(psiX)+cos(phiX)*sin(thetaX)*sin(psiX); ...
     -sin(thetaX)                             sin(phiX)*cos(thetaX)                             cos(phiX)*cos(thetaX)];  
RMATD=[cos(0)*cos(dX) -cos(0)*sin(dX)+sin(0)*sin(0)*cos(dX)  sin(0)*sin(dX)+cos(0)*sin(0)*cos(dX); ...
      cos(0)*sin(dX)  cos(0)*cos(dX)+sin(0)*sin(0)*sin(dX) -sin(0)*cos(dX)+cos(0)*sin(0)*sin(dX); ...
     -sin(0)                             sin(0)*cos(0)                             cos(0)*cos(0)];  


%Rotating the vertices to put in ship coordinate
for i=1:ntri 
    V1=[vert1(i,1); vert1(i,2); vert1(i,3);];
    V2=[vert2(i,1); vert2(i,2); vert2(i,3);];
    V3=[vert3(i,1); vert3(i,2); vert3(i,3);];
        
    %rotating to local z coordinate
    V1_o=inv(RMATX)*(V1-origin*70.2+xcg);
    V2_o=inv(RMATX)*(V2-origin*70.2+xcg);
    V3_o=inv(RMATX)*(V3-origin*70.2+xcg);
    
    %rotating for corresponding appendage deflection
    V1_x=RMATD*V1_o;
    V2_x=RMATD*V2_o;
    V3_x=RMATD*V3_o;
    
        %re-positioning the appendage to local vectors
    V1_r=RMATX*V1_x;
    V2_r=RMATX*V2_x;
    V3_r=RMATX*V3_x;
    
    %re-assigning vertices
    
    for j=1:3
    vert1(i,j)=V1_r(j)+origin(j)*70.2-xcg(j);
    vert2(i,j)=V2_r(j)+origin(j)*70.2-xcg(j);
    vert3(i,j)=V3_r(j)+origin(j)*70.2-xcg(j);
    end  
end

 
%position of mid points in earth coordinate;
mp1=zeros(ntri,3);
mp2=zeros(ntri,3);
mp3=zeros(ntri,3);
nA =zeros(ntri,3);

P1=zeros(ntri,1);
P2=zeros(ntri,1);
P3=zeros(ntri,1);

%position vector of mid points from the CG
r1=zeros(ntri,3);
r2=zeros(ntri,3);
r3=zeros(ntri,3);

v1_w=zeros(ntri,3);
v2_w=zeros(ntri,3);
v3_w=zeros(ntri,3);
n_w=zeros(ntri,3);

%Area of triangle, product of area and unit normal, position vector to each mid-point

for i=1:ntri
    %Area of each triangle
    A=[vert2(i,1)-vert1(i,1); vert2(i,2)-vert1(i,2); vert2(i,3)-vert1(i,3);];
    B=[vert3(i,1)-vert1(i,1); vert3(i,2)-vert1(i,2); vert3(i,3)-vert1(i,3);];
    C=[normal(i,1); normal(i,2); normal(i,3);];

    
    %A*n vector calculation
    for j=1:3
        nA(i,j)=dA(i).*C(j);    
    end
    
    %position vector to each mid point of each edge
    for j=1:3
        r1(i,j)=0.5*(vert1(i,j)+vert2(i,j));
        r2(i,j)=0.5*(vert1(i,j)+vert3(i,j));
        r3(i,j)=0.5*(vert2(i,j)+vert3(i,j));
    end
end

%computing mid point location between vertices in earth coordinate
for i=1:ntri
    MP1=RMat*[r1(i,1); r1(i,2); r1(i,3);]+[x_e; y_e; z_e;];
    MP2=RMat*[r2(i,1); r2(i,2); r2(i,3);]+[x_e; y_e; z_e;];
    MP3=RMat*[r3(i,1); r3(i,2); r3(i,3);]+[x_e; y_e; z_e;];
    
    v1i=RMat*[vert1(i,1); vert1(i,2); vert1(i,3);]+[x_e; y_e; z_e;];
    v2i=RMat*[vert2(i,1); vert2(i,2); vert2(i,3);]+[x_e; y_e; z_e;];
    v3i=RMat*[vert3(i,1); vert3(i,2); vert3(i,3);]+[x_e; y_e; z_e;];
    
    for j=1:3
        v1_w(i,j)=v1i(j); v2_w(i,j)=v2i(j); v3_w(i,j)=v3i(j);
        mp1(i,j)=MP1(j);  mp2(i,j)=MP2(j);  mp3(i,j)=MP3(j);
    end
end

for i=1:ntri
    A=[v2_w(i,1)-v1_w(i,1); v2_w(i,2)-v1_w(i,2); v2_w(i,3)-v1_w(i,3);];
    B=[v3_w(i,1)-v1_w(i,1); v3_w(i,2)-v1_w(i,2); v3_w(i,3)-v1_w(i,3);];
    n=cross(A,B)/norm(cross(A,B));
    dA(i,1)=0.5*norm(cross(A,B));
    n_w(i,1)=n(1); n_w(i,2)=n(2); n_w(i,3)=n(3);
end

if fwrite==1
if rem(time,its)==0
%writing the transformed surface grid
filename=['./SurfOut/X2_2_' sprintf('%08.2f',time) '.stl'];
fileID = fopen(filename,'w');
formatSpec='solid\n'; fprintf(fileID,formatSpec);
for i=1:ntri
fprintf(fileID,'facet normal ');
formatSpec='%1.8e %1.8e %1.8e\n';
fprintf(fileID,formatSpec,normal(i,1),normal(i,2),normal(i,3));
    fprintf(fileID,'  outer loop\n')
    fprintf(fileID,'    vertex   ')
    fprintf(fileID,formatSpec,v1_w(i,1)/70.2,v1_w(i,2)/70.2,v1_w(i,3)/70.2)
    fprintf(fileID,'    vertex   ')
    fprintf(fileID,formatSpec,v2_w(i,1)/70.2,v2_w(i,2)/70.2,v2_w(i,3)/70.2)
    fprintf(fileID,'    vertex   ')
    fprintf(fileID,formatSpec,v3_w(i,1)/70.2,v3_w(i,2)/70.2,v3_w(i,3)/70.2)
    fprintf(fileID,'  endloop\n')
    fprintf(fileID,'endfacet\n')
end
formatSpec='endsolid'; fprintf(fileID,formatSpec);
fclose(fileID);
end
end

%computing forces and moments for each triangle
Fx_total=0; Fy_total=0; Fz_total=0;
Mx_total=0; My_total=0; Mz_total=0;

for i=1:ntri
    p1=-rho*g*(mp1(i,3)-A_wave*exp(k_wave.*mp1(i,3)).*sin(k_wave*mp1(i,1)-w_wave.*time));
    p2=-rho*g*(mp2(i,3)-A_wave*exp(k_wave.*mp2(i,3)).*sin(k_wave*mp2(i,1)-w_wave.*time));
    p3=-rho*g*(mp3(i,3)-A_wave*exp(k_wave.*mp3(i,3)).*sin(k_wave*mp3(i,1)-w_wave.*time));
    
    dFx=-nA(i,1)*(p1+p2+p3)./3;
    dFy=-nA(i,2)*(p1+p2+p3)./3;
    dFz=-nA(i,3)*(p1+p2+p3)./3;
    
    dP =-p1.*[r1(i,1); r1(i,2); r1(i,3)-Zb;]...
        -p2.*[r2(i,1); r2(i,2); r2(i,3)-Zb;]...
        -p3.*[r3(i,1); r3(i,2); r3(i,3)-Zb;];
    N =[nA(i,1); nA(i,2); nA(i,3);];
    dM=cross(dP,N);
    Fx_total=Fx_total+dFx;
    Fy_total=Fy_total+dFy;
    Fz_total=Fz_total+dFz;
    Mx_total=Mx_total+dM(1)/3;
    My_total=My_total+dM(2)/3;
    Mz_total=Mz_total+dM(3)/3;
end
end

== matlab function Model_6DOF_B3/HDM B3/Wave, Virtual Mass and Hydrostatic/Wave Particle Motions/Subsystem/X2/MATLAB Function4 ==
  data: time input; Xearth input; Fx_total output; vert1 input; vert2 input; vert3 input; dA input; ntri input; normal input; A_wave input; k_wave input; w_wave input; rho input; g input; Fy_total output; Fz_total output; Mx_total output; My_total output; Mz_total output; Zb input; EAX input; dX input; its input; origin input; xcg input; fwrite input
function [Fx_total,Fy_total,Fz_total,Mx_total,My_total,Mz_total]= fcn(time,Xearth,vert1,vert2,vert3,dA,ntri,normal,A_wave,k_wave,w_wave,rho,g,Zb,EAX,dX,its,origin,xcg,fwrite)
%EAX=Appendage eulater angle in local coordinate
%its=number of time steps to skip writing grid

x_e=Xearth(1); y_e=Xearth(2); z_e=Xearth(3);
phi=Xearth(4); theta=Xearth(5); psi=Xearth(6);
phiX=EAX(1); thetaX=EAX(2); psiX=EAX(3);


RMat=[cos(theta)*cos(psi) -cos(phi)*sin(psi)+sin(phi)*sin(theta)*cos(psi)  sin(phi)*sin(psi)+cos(phi)*sin(theta)*cos(psi); ...
      cos(theta)*sin(psi)  cos(phi)*cos(psi)+sin(phi)*sin(theta)*sin(psi) -sin(phi)*cos(psi)+cos(phi)*sin(theta)*sin(psi); ...
     -sin(theta)                             sin(phi)*cos(theta)                             cos(phi)*cos(theta)];  
RMATX=[cos(thetaX)*cos(psiX) -cos(phiX)*sin(psiX)+sin(phiX)*sin(thetaX)*cos(psiX)  sin(phiX)*sin(psiX)+cos(phiX)*sin(thetaX)*cos(psiX); ...
      cos(thetaX)*sin(psiX)  cos(phiX)*cos(psiX)+sin(phiX)*sin(thetaX)*sin(psiX) -sin(phiX)*cos(psiX)+cos(phiX)*sin(thetaX)*sin(psiX); ...
     -sin(thetaX)                             sin(phiX)*cos(thetaX)                             cos(phiX)*cos(thetaX)];  
RMATD=[cos(0)*cos(dX) -cos(0)*sin(dX)+sin(0)*sin(0)*cos(dX)  sin(0)*sin(dX)+cos(0)*sin(0)*cos(dX); ...
      cos(0)*sin(dX)  cos(0)*cos(dX)+sin(0)*sin(0)*sin(dX) -sin(0)*cos(dX)+cos(0)*sin(0)*sin(dX); ...
     -sin(0)                             sin(0)*cos(0)                             cos(0)*cos(0)];  


%Rotating the vertices to put in ship coordinate
for i=1:ntri 
    V1=[vert1(i,1); vert1(i,2); vert1(i,3);];
    V2=[vert2(i,1); vert2(i,2); vert2(i,3);];
    V3=[vert3(i,1); vert3(i,2); vert3(i,3);];
        
    %rotating to local z coordinate
    V1_o=inv(RMATX)*(V1-origin*70.2+xcg);
    V2_o=inv(RMATX)*(V2-origin*70.2+xcg);
    V3_o=inv(RMATX)*(V3-origin*70.2+xcg);
    
    %rotating for corresponding appendage deflection
    V1_x=RMATD*V1_o;
    V2_x=RMATD*V2_o;
    V3_x=RMATD*V3_o;
    
        %re-positioning the appendage to local vectors
    V1_r=RMATX*V1_x;
    V2_r=RMATX*V2_x;
    V3_r=RMATX*V3_x;
    
    %re-assigning vertices
    
    for j=1:3
    vert1(i,j)=V1_r(j)+origin(j)*70.2-xcg(j);
    vert2(i,j)=V2_r(j)+origin(j)*70.2-xcg(j);
    vert3(i,j)=V3_r(j)+origin(j)*70.2-xcg(j);
    end  
end

 
%position of mid points in earth coordinate;
mp1=zeros(ntri,3);
mp2=zeros(ntri,3);
mp3=zeros(ntri,3);
nA =zeros(ntri,3);

P1=zeros(ntri,1);
P2=zeros(ntri,1);
P3=zeros(ntri,1);

%position vector of mid points from the CG
r1=zeros(ntri,3);
r2=zeros(ntri,3);
r3=zeros(ntri,3);

v1_w=zeros(ntri,3);
v2_w=zeros(ntri,3);
v3_w=zeros(ntri,3);
n_w=zeros(ntri,3);

%Area of triangle, product of area and unit normal, position vector to each mid-point

for i=1:ntri
    %Area of each triangle
    A=[vert2(i,1)-vert1(i,1); vert2(i,2)-vert1(i,2); vert2(i,3)-vert1(i,3);];
    B=[vert3(i,1)-vert1(i,1); vert3(i,2)-vert1(i,2); vert3(i,3)-vert1(i,3);];
    C=[normal(i,1); normal(i,2); normal(i,3);];

    
    %A*n vector calculation
    for j=1:3
        nA(i,j)=dA(i).*C(j);    
    end
    
    %position vector to each mid point of each edge
    for j=1:3
        r1(i,j)=0.5*(vert1(i,j)+vert2(i,j));
        r2(i,j)=0.5*(vert1(i,j)+vert3(i,j));
        r3(i,j)=0.5*(vert2(i,j)+vert3(i,j));
    end
end

%computing mid point location between vertices in earth coordinate
for i=1:ntri
    MP1=RMat*[r1(i,1); r1(i,2); r1(i,3);]+[x_e; y_e; z_e;];
    MP2=RMat*[r2(i,1); r2(i,2); r2(i,3);]+[x_e; y_e; z_e;];
    MP3=RMat*[r3(i,1); r3(i,2); r3(i,3);]+[x_e; y_e; z_e;];
    
    v1i=RMat*[vert1(i,1); vert1(i,2); vert1(i,3);]+[x_e; y_e; z_e;];
    v2i=RMat*[vert2(i,1); vert2(i,2); vert2(i,3);]+[x_e; y_e; z_e;];
    v3i=RMat*[vert3(i,1); vert3(i,2); vert3(i,3);]+[x_e; y_e; z_e;];
    
    for j=1:3
        v1_w(i,j)=v1i(j); v2_w(i,j)=v2i(j); v3_w(i,j)=v3i(j);
        mp1(i,j)=MP1(j);  mp2(i,j)=MP2(j);  mp3(i,j)=MP3(j);
    end
end

for i=1:ntri
    A=[v2_w(i,1)-v1_w(i,1); v2_w(i,2)-v1_w(i,2); v2_w(i,3)-v1_w(i,3);];
    B=[v3_w(i,1)-v1_w(i,1); v3_w(i,2)-v1_w(i,2); v3_w(i,3)-v1_w(i,3);];
    n=cross(A,B)/norm(cross(A,B));
    dA(i,1)=0.5*norm(cross(A,B));
    n_w(i,1)=n(1); n_w(i,2)=n(2); n_w(i,3)=n(3);
end

if fwrite==1
if rem(time,its)==0
%writing the transformed surface grid
filename=['./SurfOut/X2_1_' sprintf('%08.2f',time) '.stl'];
fileID = fopen(filename,'w');
formatSpec='solid\n'; fprintf(fileID,formatSpec);
for i=1:ntri
fprintf(fileID,'facet normal ');
formatSpec='%1.8e %1.8e %1.8e\n';
fprintf(fileID,formatSpec,normal(i,1),normal(i,2),normal(i,3));
    fprintf(fileID,'  outer loop\n')
    fprintf(fileID,'    vertex   ')
    fprintf(fileID,formatSpec,v1_w(i,1)/70.2,v1_w(i,2)/70.2,v1_w(i,3)/70.2)
    fprintf(fileID,'    vertex   ')
    fprintf(fileID,formatSpec,v2_w(i,1)/70.2,v2_w(i,2)/70.2,v2_w(i,3)/70.2)
    fprintf(fileID,'    vertex   ')
    fprintf(fileID,formatSpec,v3_w(i,1)/70.2,v3_w(i,2)/70.2,v3_w(i,3)/70.2)
    fprintf(fileID,'  endloop\n')
    fprintf(fileID,'endfacet\n')
end
formatSpec='endsolid'; fprintf(fileID,formatSpec);
fclose(fileID);
end
end

%computing forces and moments for each triangle
Fx_total=0; Fy_total=0; Fz_total=0;
Mx_total=0; My_total=0; Mz_total=0;

for i=1:ntri
    p1=-rho*g*(mp1(i,3)-A_wave*exp(k_wave.*mp1(i,3)).*sin(k_wave*mp1(i,1)-w_wave.*time));
    p2=-rho*g*(mp2(i,3)-A_wave*exp(k_wave.*mp2(i,3)).*sin(k_wave*mp2(i,1)-w_wave.*time));
    p3=-rho*g*(mp3(i,3)-A_wave*exp(k_wave.*mp3(i,3)).*sin(k_wave*mp3(i,1)-w_wave.*time));
    
    dFx=-nA(i,1)*(p1+p2+p3)./3;
    dFy=-nA(i,2)*(p1+p2+p3)./3;
    dFz=-nA(i,3)*(p1+p2+p3)./3;
    
    dP =-p1.*[r1(i,1); r1(i,2); r1(i,3)-Zb;]...
        -p2.*[r2(i,1); r2(i,2); r2(i,3)-Zb;]...
        -p3.*[r3(i,1); r3(i,2); r3(i,3)-Zb;];
    N =[nA(i,1); nA(i,2); nA(i,3);];
    dM=cross(dP,N);
    Fx_total=Fx_total+dFx;
    Fy_total=Fy_total+dFy;
    Fz_total=Fz_total+dFz;
    Mx_total=Mx_total+dM(1)/3;
    My_total=My_total+dM(2)/3;
    Mz_total=Mz_total+dM(3)/3;
end
end

== matlab function Model_6DOF_B3/HDM 6DOF V1/Y/Fy ==
  data: Bx input; Bv input; Ba input; CYr input; CYvr input; CYrr input; CYuvw input; Umag input; UeX input; dLCG input; dmass input; CYdXi input; Mb parameter; Bb parameter; Fy output; FYr output; FYx1 output; FYx2 output; FYx3 output; FYx4 output; FYuvw output; FYhull output; FYApp output; Yvm input
 function [Fy,FYr,FYx1,FYx2,FYx3,FYx4,FYuvw,FYhull,FYApp]  = fcn(Bx,Bv,Ba,CYr,CYvr,CYrr,CYuvw,Umag,UeX,dLCG,dmass,CYdXi,Mb,Bb,Yvm)
%Bx,Bv,Ba are the body motion position, velocity, acceleration in ship coordinate
%Wv,Wa are the wave particle velocity, acceleration in ship coordinate
 
u=Bv(1); v=Bv(2); w=Bv(3); p=Bv(4); q=Bv(5); r=Bv(6);
x=Bx(1); y=Bx(2); z=Bx(3); phi=Bx(4); theta=Bx(5); psi=Bx(6);
a1=Ba(1); a2=Ba(2); a3=Ba(3); a4=Ba(4); a5=Ba(5); a6=Ba(6); 

FYuvw=0.5*1025*70.2^2*CYuvw*Umag^2

FYx1=1025*70.2^2*CYdXi(1)*UeX(1)^2
FYx2=1025*70.2^2*CYdXi(2)*UeX(2)^2
FYx3=1025*70.2^2*CYdXi(3)*UeX(3)^2
FYx4=1025*70.2^2*CYdXi(4)*UeX(4)^2

FYrr=0.5*1025*70.2^4*CYrr*q*abs(q)*0
FYr =1025*70.2^2*(0.9*8.2086E-03*u*r)*u^2*2

%FYr =0.5*1025*70.2^3*CYr*u^2*2
FYvr=0.5*1025*70.2^3*CYvr*u^2*0

FYhull=FYuvw+FYr+FYvr+FYrr
FYApp=FYx1+FYx2+FYx3+FYx4
FYStat=((Mb+dmass)-Bb)*9.81*cos(theta)*sin(phi)

Fy=FYApp+FYStat+FYhull+Yvm
 end
